simulink library "ddm"  (R2021b)
settings: Solver=VariableStepAuto  StartTime=0.0  StopTime=10.0  RelTol=1e-3
undefined symbols (not defined in the file or in its folder): ENUM_ADASACCSTA_ERROR, ENUM_ADASACCSTA_OFF, ENUM_ADASACCSTA_STANDBY, ENUM_ADASISASTA_OFF, ENUM_ALLOWMOV_ALLOWREADY, ENUM_APS, ENUM_BRKSTA_ERROR, ENUM_BRKSTA_OFF, ENUM_BRKSTA_ON, ENUM_BRKSW_INVALID, ENUM_BRKSW_OFF, ENUM_BRKSW_ON, ENUM_CHGPREACTERRSTA_OBCPRE, ENUM_DCDCFAULTSTA_ANYFAULTLV1, ENUM_DCDCFAULTSTA_ANYFAULTLV2, ENUM_DRIVETRAIN_AWD, ENUM_DRIVETRAIN_FWD, ENUM_DRIVETRAIN_RWD, ENUM_DRSEATSTA_INVALID, ENUM_EDUDRTSTA_NORMAL, ENUM_EPBSTA_APPLIED, ENUM_EPBSTA_RELEASED, ENUM_HVBATTREADYPRE_READY, ENUM_MCUWARN_LV0, ENUM_MCUWARN_LV1, ENUM_MCUWARN_LV2, ENUM_MCUWARN_LV3, ENUM_MCUWARN_NOERROR, ENUM_OBCFAULTSTA_ANYFAULT, ENUM_PAS_R2F2, ENUM_PDFAULT_BATTPDFAIL, ENUM_PDFAULT_DCDCDISABLE, ENUM_PDFAULT_MCUDISABLE, ENUM_PDFAULT_MCUDISCHRG, ENUM_POWERSTA_OFF, ENUM_POWERSTA_ON, ENUM_POWERSTA_READY, ENUM_POWERSTA_STANDBY, ENUM_PRESSINDI_LOW, ENUM_PUFAULT_BATTUPFAIL, ENUM_PUFAULT_DCDCENABLEFAIL, ENUM_PUFAULT_PRECHRGCHKFAIL, ENUM_PUFAULT_SAFETYCHKFAIL, ENUM_PUSTATE_COMPLETED, ENUM_PWRSTASW_OFF, ENUM_PWRSTASW_OFFA, ENUM_PWRSTASW_OFFCHVCHRG, ENUM_PWRSTASW_OFFCLVCHRG, ENUM_PWRSTASW_ON, ENUM_PWRSTASW_ONHVCHRG, ENUM_PWRSTASW_READY, ENUM_PWRSTASW_STANDBY, ENUM_RANGESTA_12IN, ENUM_SHIFTCOMMAND_D, ENUM_SHIFTCOMMAND_N, ENUM_SHIFTCOMMAND_P, ENUM_SHIFTCOMMAND_R, ENUM_VEHMALFUNLV_2ND, ENUM_VEHMALFUNLV_3RD, ENUM_VEHMALFUNLV_4TH ... (+835)
libraries: hcu_lib x750, $bdroot x12, simulink x5
(part 21 of 28)

== system ddm/DDM/DDM/PMM/power up and power down/BMS ready fail ==
  note: Diagnostics and Fault Handling
  note: Release Condition After Failure Decision
  note: Test Detection Criteria
  note: Test Pass Criteria
  note: Release Condition During Failure Detection
  note: Fail Safe Operation During Failure Detection
  note: Fail Safe Operation After Failure Decision
  task_time_s : Inport
  VPMM_PowerSta_enum : Inport  Port=2
  VPMM_PwrStaSW_enum : Inport  Port=3
  VINP_BMSREADY_flg : Inport  Port=4
  VPMM_PowerUpFault_enum : Inport  Port=5
  DTC_clear_request : Inport  Port=6
  VPMM_PowerUpState_enum : Inport  Port=7
  Constant : Constant  Value=ENUM_PUFAULT_BATTUPFAIL
  Constant1 : Constant  Value=ENUM_PWRSTASW_OFF
  Constant10 : Constant  Value=KDDM_BMSRdyDTC_cnt
  Constant11 : Constant  Value=KDDM_BMSRdyPassSW_flg
  Constant15 : Constant  Value=KDDM_BMSRdyCFSSW_flg
  Constant16 : Constant  Value=TRUE
  Constant19 : Constant  Value=ENUM_POWERSTA_OFF
  Constant2 : Constant  Value=ENUM_PUSTATE_COMPLETED
  Constant20 : Constant  Value=KDDM_BMSRdyDFSSW_flg
  Constant{3,21,25,27} (4 alike) : Constant  Value=FALSE
  Constant23 : Constant  Value=TRUE
  Constant24 : Constant  Value=TRUE
  Constant38 : Constant  Commented=on  Value=KDDM_BMSRdyDetTO_s
  Constant40 : Constant  Commented=on  Value=KDDM_BMSRdyDTC_cnt
  Constant43 : Constant  Value=KDDM_BMSRdyPassTO_s
  Constant44 : Constant  Value=KDDM_BMSRdyDetSW_flg
  Constant8 : Constant  Value=KDDM_BMSRdyPassTO_s
  DTC_Couter : hcu_lib/Basic_Blocks/DTC_Couter
  DTC_Info : hcu_lib/Basic_Blocks/DTC_Info
  Data Type Conversion1 : DataTypeConversion  OutDataTypeStr=uint8
  Equal : RelationalOperator  Operator=~=  OutDataTypeStr=boolean  RndMeth=Simplest
  Equal1 : RelationalOperator  Operator===  OutDataTypeStr=boolean  RndMeth=Simplest
  Equal2 : RelationalOperator  Operator===  OutDataTypeStr=boolean  RndMeth=Simplest
  Equal5 : RelationalOperator  OutDataTypeStr=boolean  RndMeth=Simplest
  Equal6 : RelationalOperator  Operator===  OutDataTypeStr=boolean  RndMeth=Simplest
  From48 : From  Commented=on  GotoTag=task_time_s
  Goto24 : Goto  Commented=on  GotoTag=VDDM_EDriveSysErrVCUErr_flg
  Logical Operator1 : Logic  Operator=OR  AllPortsSameDT=off  OutDataTypeStr=boolean
  Logical Operator{5,12,15,18} (4 alike) : Logic  AllPortsSameDT=off  OutDataTypeStr=boolean
  Logical Operator19 : Logic  Inputs=3  AllPortsSameDT=off  OutDataTypeStr=boolean
  Logical Operator2 : Logic  Operator=NOT  AllPortsSameDT=off  OutDataTypeStr=boolean
  Logical Operator3 : Logic  Operator=OR  Inputs=3  AllPortsSameDT=off  OutDataTypeStr=boolean
  Logical Operator4 : Logic  Operator=NOT  AllPortsSameDT=off  OutDataTypeStr=boolean
  Logical Operator6 : Logic  Operator=NOT  AllPortsSameDT=off  OutDataTypeStr=boolean
  Logical Operator7 : Logic  Operator=OR  AllPortsSameDT=off  OutDataTypeStr=boolean
  Logical Operator8 : Logic  Operator=OR  AllPortsSameDT=off  OutDataTypeStr=boolean
  Relay : Relay  OnSwitchValue=ONE_INT  OffSwitchValue=ZERO_INT
  SR_Latch1 : Subsystem  mask(SR_Latch){}
      mask help: SR latch function.
  SR_Latch3 : hcu_lib/Basic_Blocks/SR_Latch
  SR_Latch4 : hcu_lib/Basic_Blocks/SR_Latch
  Switch{,2,4..5} (4 alike) : Switch  Criteria=u2 ~= 0
  Test Detection Criteria : hcu_lib/Basic_Blocks/Test Detection Criteria  Commented=on
  Timer1 : hcu_lib/Basic_Blocks/Timer
  VDDM_BMSRdyDTC_raw32 : Outport
  wires:
  [DTC_clear_request] -> Logical Operator7/2
  Logical Operator7/1 -> SR_Latch3/2
  Logical Operator1/1 -> SR_Latch4/2
  Logical Operator2/1 -> Logical Operator19/3
  [DTC_clear_request] -> Logical Operator3/3
  Logical Operator12/1 -> [VDDM_BMSRdyDFS_flg]  "VDDM_BMSRdyDFS_flg"
  Logical Operator18/1 -> [VDDM_BMSRdyCFS_flg]  "VDDM_BMSRdyCFS_flg"
  [VDDM_BMSRdyCFS_flg] -> Logical Operator7/1
  Data Type Conversion1/1 -> [VDDM_BMSRdyDTC_cnt]  "VDDM_BMSRdyDTC_cnt"
  Logical Operator15/1 -> DTC_Couter/2
  [VDDM_BMSRdyPass_flg] -> Logical Operator3/1
  [DTC_clear_request] -> Logical Operator2/1
  [VDDM_BMSRdyDet_flg] -> Logical Operator19/1
  DTC_Couter/1 -> SR_Latch4/1
  Constant20/1 -> Logical Operator12/1
  Constant15/1 -> Logical Operator18/2
  [DTC_clear_request] -> Logical Operator1/2
  Constant10/1 -> DTC_Couter/3
  Logical Operator19/1 -> DTC_Couter/1
  SR_Latch4/1 -> Logical Operator18/1
  Relay/1 -> SR_Latch3/1
  SR_Latch3/1 -> Logical Operator12/2
  Constant44/1 -> Logical Operator19/2
  [VDDM_BMSRdyCFSRls_flg] -> Logical Operator3/2
  [VDDM_BMSRdyDTC_cnt] -> Relay/1
  [VDDM_BMSRdyCFSRls_flg] -> Logical Operator1/1
  Constant11/1 -> Logical Operator15/2
  Logical Operator3/1 -> Logical Operator15/1
  DTC_Couter/2 -> Data Type Conversion1/1
  [VPMM_PowerUpState_enum] -> Equal2/1
  Constant2/1 -> Equal2/2
  Constant3/1 -> Switch2/1
  VPMM_PowerUpState_enum/1 -> [VPMM_PowerUpState_enum]
  [DTC_clear_request] -> DTC_Info/4
  Constant38/1 -> Test Detection Criteria/4
  [VDDM_BMSRdyPass_flg] -> DTC_Info/2
  [VDDM_BMSRdyDet_flg] -> DTC_Info/1
  [VDDM_BMSRdyCFS_flg] -> DTC_Info/3
  DTC_Info/1 -> VDDM_BMSRdyDTC_raw32/1  "VDDM_BMSRdyDTC_raw32"
  task_time_s/1 -> [task_time_s]
  VPMM_PwrStaSW_enum/1 -> [VPMM_PwrStaSW_enum]
  VPMM_PowerSta_enum/1 -> [VPMM_PowerSta_enum]
  Constant21/1 -> Switch/3
  Equal5/1 -> SR_Latch1/1(set)
  Switch4/1 -> [VDDM_BMSRdyCFSRls_flg]  "VDDM_BMSRdyCFSRls_flg"
  Constant8/1 -> Equal5/2
  [task_time_s] -> Timer1/3
  [VPMM_PowerSta_enum] -> Equal6/1
  Constant23/1 -> Switch2/3
  Constant16/1 -> Switch/1
  Constant1/1 -> Equal/2
  From48/1 -> Test Detection Criteria/2
  Switch/1 -> Goto24/1
  Switch5/1 -> [VDDM_BMSRdyDet_flg]  "VDDM_BMSRdyDet_flg"
  Constant24/1 -> Switch4/1
  Constant40/1 -> Test Detection Criteria/3
  Constant25/1 -> Switch4/3
  [VPMM_PwrStaSW_enum] -> Equal/1
  [VDDM_BMSRdyCFS_flg] -> Switch/2
  [DTC_clear_request] -> Logical Operator8/2
  Equal2/1 -> Switch2/2
  Equal/1 -> Switch5/2
  Logical Operator8/1 -> Switch4/2
  Logical Operator6/1 -> Timer1/1
  SR_Latch1/1(latched) -> [VDDM_BMSRdyPass_flg]  "VDDM_BMSRdyPass_flg"
  Equal6/1 -> Logical Operator8/1
  Constant27/1 -> Switch5/3
  Constant43/1 -> Timer1/4
  Constant19/1 -> Equal6/2
  [VDDM_BMSRdyChk_flg] -> Switch5/1
  Timer1/1 -> Equal5/1
  Switch2/1 -> SR_Latch1/2(reset), Timer1/2, Logical Operator6/1
  DTC_clear_request/1 -> [DTC_clear_request]
  Constant/1 -> Equal1/2
  Equal1/1 -> Logical Operator5/2
  Logical Operator4/1 -> Logical Operator5/1
  VINP_BMSREADY_flg/1 -> Logical Operator4/1
  VPMM_PowerUpFault_enum/1 -> Equal1/1
  Logical Operator5/1 -> [VDDM_BMSRdyChk_flg]

== system ddm/DDM/DDM/PMM/power up and power down/DCDC disable fail ==
  note: Diagnostics and Fault Handling
  note: Test Pass Criteria
  note: Test Detection Criteria
  note: Release Condition During Failure Detection
  note: Release Condition After Failure Decision
  note: Fail Safe Operation During Failure Detection
  note: Fail Safe Operation After Failure Decision
  task_time_s : Inport
  VPMM_PowerSta_enum : Inport  Port=2
  VPMM_PwrStaSW_enum : Inport  Port=3
  VPMM_PowerDownFault_enum : Inport  Port=4
  DTC_clear_request : Inport  Port=5
  Constant : Constant  Value=ENUM_PDFAULT_DCDCDISABLE
  Constant1 : Constant  Value=ENUM_PWRSTASW_OFF
  Constant10 : Constant  Value=KDDM_DCDCDisDTC_cnt
  Constant11 : Constant  Value=KDDM_DCDCDisPassSW_flg
  Constant15 : Constant  Value=KDDM_DCDCDisCFSSW_flg
  Constant16 : Constant  Value=TRUE
  Constant17 : Constant  Value=KDDM_DCDCDisPassTO_s
  Constant19 : Constant  Value=ENUM_POWERSTA_OFF
  Constant20 : Constant  Value=KDDM_DCDCDisDFSSW_flg
  Constant21 : Constant  Value=FALSE
  Constant22 : Constant  Value=ENUM_PWRSTASW_OFF
  Constant23 : Constant  Value=TRUE
  Constant24 : Constant  Value=TRUE
  Constant25 : Constant  Value=FALSE
  Constant27 : Constant  Value=FALSE
  Constant38 : Constant  Commented=on  Value=KDDM_DCDCDisDetTO_s
  Constant40 : Constant  Commented=on  Value=KDDM_DCDCDisDTC_cnt
  Constant43 : Constant  Value=KDDM_DCDCDisPassTO_s
  Constant44 : Constant  Value=KDDM_DCDCDisDetSW_flg
  DTC_Couter : hcu_lib/Basic_Blocks/DTC_Couter
  DTC_Info : hcu_lib/Basic_Blocks/DTC_Info
  Data Type Conversion1 : DataTypeConversion  OutDataTypeStr=uint8
  Equal1 : RelationalOperator  Operator===  OutDataTypeStr=boolean  RndMeth=Simplest
  Equal2 : RelationalOperator  Operator=~=  OutDataTypeStr=boolean  RndMeth=Simplest
  Equal4 : RelationalOperator  Operator=~=  OutDataTypeStr=boolean  RndMeth=Simplest
  Equal6 : RelationalOperator  OutDataTypeStr=boolean  RndMeth=Simplest
  Equal7 : RelationalOperator  Operator===  OutDataTypeStr=boolean  RndMeth=Simplest
  From48 : From  Commented=on  GotoTag=task_time_s
  Goto24 : Goto  Commented=on  GotoTag=VDDM_EDriveSysErrVCUErr_flg
  Logical Operator1 : Logic  Operator=NOT  AllPortsSameDT=off  OutDataTypeStr=boolean
  Logical Operator12 : Logic  AllPortsSameDT=off  OutDataTypeStr=boolean
  Logical Operator15 : Logic  AllPortsSameDT=off  OutDataTypeStr=boolean
  Logical Operator18 : Logic  AllPortsSameDT=off  OutDataTypeStr=boolean
  Logical Operator19 : Logic  Inputs=3  AllPortsSameDT=off  OutDataTypeStr=boolean
  Logical Operator2 : Logic  Operator=OR  AllPortsSameDT=off  OutDataTypeStr=boolean
  Logical Operator3 : Logic  Operator=OR  Inputs=3  AllPortsSameDT=off  OutDataTypeStr=boolean
  Logical Operator4 : Logic  Operator=OR  AllPortsSameDT=off  OutDataTypeStr=boolean
  Logical Operator6 : Logic  Operator=NOT  AllPortsSameDT=off  OutDataTypeStr=boolean
  Logical Operator8 : Logic  Operator=OR  AllPortsSameDT=off  OutDataTypeStr=boolean
  Relay : Relay  OnSwitchValue=ONE_INT  OffSwitchValue=ZERO_INT
  SR_Latch1 : Subsystem  mask(SR_Latch){}
      mask help: SR latch function.
  SR_Latch3 : hcu_lib/Basic_Blocks/SR_Latch
  SR_Latch4 : hcu_lib/Basic_Blocks/SR_Latch
  Switch{,1,4..5} (4 alike) : Switch  Criteria=u2 ~= 0
  Test Detection Criteria : hcu_lib/Basic_Blocks/Test Detection Criteria  Commented=on
  Timer1 : hcu_lib/Basic_Blocks/Timer
  VDDM_DCDCDisDTC_raw32 : Outport
  wires:
  [VDDM_DCDCDisDet_flg] -> Logical Operator19/1
  [DTC_clear_request] -> Logical Operator3/3
  DTC_Couter/2 -> Data Type Conversion1/1
  Logical Operator2/1 -> SR_Latch4/2
  Logical Operator1/1 -> Logical Operator19/3
  [DTC_clear_request] -> Logical Operator1/1
  Relay/1 -> SR_Latch3/1
  Constant20/1 -> Logical Operator12/1
  [VDDM_DCDCDisCFSRls_flg] -> Logical Operator2/1
  SR_Latch4/1 -> Logical Operator18/1
  [VDDM_DCDCDisCFS_flg] -> Logical Operator4/1
  [VDDM_DCDCDisDTC_cnt] -> Relay/1
  Logical Operator3/1 -> Logical Operator15/1
  Logical Operator18/1 -> [VDDM_DCDCDisCFS_flg]  "VDDM_DCDCDisCFS_flg"
  Constant11/1 -> Logical Operator15/2
  Constant10/1 -> DTC_Couter/3
  [VDDM_DCDCDisPass_flg] -> Logical Operator3/1
  [DTC_clear_request] -> Logical Operator4/2
  Constant44/1 -> Logical Operator19/2
  Logical Operator15/1 -> DTC_Couter/2
  [DTC_clear_request] -> Logical Operator2/2
  SR_Latch3/1 -> Logical Operator12/2
  [VDDM_DCDCDisCFSRls_flg] -> Logical Operator3/2
  Logical Operator19/1 -> DTC_Couter/1
  Logical Operator12/1 -> [VDDM_DCDCDisDFS_flg]  "VDDM_DCDCDisDFS_flg"
  Constant15/1 -> Logical Operator18/2
  Data Type Conversion1/1 -> [VDDM_DCDCDisDTC_cnt]  "VDDM_DCDCDisDTC_cnt"
  DTC_Couter/1 -> SR_Latch4/1
  Logical Operator4/1 -> SR_Latch3/2
  [DTC_clear_request] -> DTC_Info/4
  Constant38/1 -> Test Detection Criteria/4
  [VDDM_DCDCDisDet_flg] -> DTC_Info/1
  [VDDM_DCDCDisCFS_flg] -> DTC_Info/3
  [VDDM_DCDCDisPass_flg] -> DTC_Info/2
  DTC_Info/1 -> VDDM_DCDCDisDTC_raw32/1  "VDDM_DCDCDisDTC_raw32"
  Equal1/1 -> [VDDM_DCDCDisChk_flg]
  DTC_clear_request/1 -> [DTC_clear_request]
  Constant/1 -> Equal1/2
  VPMM_PowerDownFault_enum/1 -> Equal1/1
  Equal7/1 -> Logical Operator8/1
  Constant1/1 -> Equal2/2
  [VPMM_PwrStaSW_enum] -> Equal2/1
  Constant40/1 -> Test Detection Criteria/3
  [DTC_clear_request] -> Logical Operator8/2
  Timer1/1 -> Equal6/1
  [task_time_s] -> Timer1/3
  Constant22/1 -> Equal4/2
  Switch1/1 -> Timer1/2, SR_Latch1/2(reset), Logical Operator6/1
  Equal2/1 -> Switch1/2
  Equal4/1 -> Switch5/2
  [VPMM_PowerSta_enum] -> Equal7/1
  SR_Latch1/1(latched) -> [VDDM_DCDCDisPass_flg]  "VDDM_DCDCDisPass_flg"
  Constant23/1 -> Switch1/3
  [VDDM_DCDCDisChk_flg] -> Switch1/1
  [VPMM_PwrStaSW_enum] -> Equal4/1
  Constant43/1 -> Timer1/4
  Equal6/1 -> SR_Latch1/1(set)
  Constant17/1 -> Equal6/2
  Constant27/1 -> Switch5/3
  Constant25/1 -> Switch4/3
  Switch4/1 -> [VDDM_DCDCDisCFSRls_flg]  "VDDM_DCDCDisCFSRls_flg"
  Constant16/1 -> Switch/1
  [VDDM_DCDCDisCFS_flg] -> Switch/2
  [VDDM_DCDCDisChk_flg] -> Switch5/1
  Constant19/1 -> Equal7/2
  Constant21/1 -> Switch/3
  Constant24/1 -> Switch4/1
  From48/1 -> Test Detection Criteria/2
  Switch/1 -> Goto24/1
  Logical Operator8/1 -> Switch4/2
  Logical Operator6/1 -> Timer1/1
  Switch5/1 -> [VDDM_DCDCDisDet_flg]  "VDDM_DCDCDisDet_flg"
  task_time_s/1 -> [task_time_s]
  VPMM_PwrStaSW_enum/1 -> [VPMM_PwrStaSW_enum]
  VPMM_PowerSta_enum/1 -> [VPMM_PowerSta_enum]

== system ddm/DDM/DDM/PMM/power up and power down/DCDC enable fail ==
  note: Diagnostics and Fault Handling
  note: Fail Safe Operation After Failure Decision
  note: Fail Safe Operation During Failure Detection
  note: Release Condition During Failure Detection
  note: Test Pass Criteria
  note: Test Detection Criteria
  note: Release Condition After Failure Decision
  task_time_s : Inport
  VPMM_PowerSta_enum : Inport  Port=2
  VPMM_PwrStaSW_enum : Inport  Port=3
  VINP_DCDCEnabled_flg : Inport  Port=4
  VPMM_PowerUpFault_enum : Inport  Port=5
  DTC_clear_request : Inport  Port=6
  VPMM_PowerUpState_enum : Inport  Port=7
  Constant : Constant  Value=ENUM_PUFAULT_DCDCENABLEFAIL
  Constant1 : Constant  Value=ENUM_PUSTATE_COMPLETED
  Constant10 : Constant  Value=KDDM_DCDCEnaDTC_cnt
  Constant11 : Constant  Value=KDDM_DCDCEnaPassSW_flg
  Constant15 : Constant  Value=KDDM_DCDCEnaCFSSW_flg
  Constant16 : Constant  Value=TRUE
  Constant19 : Constant  Value=ENUM_POWERSTA_OFF
  Constant{2,21,25,27} (4 alike) : Constant  Value=FALSE
  Constant20 : Constant  Value=KDDM_DCDCEnaDFSSW_flg
  Constant23 : Constant  Value=TRUE
  Constant24 : Constant  Value=TRUE
  Constant26 : Constant  Value=ENUM_PWRSTASW_OFF
  Constant38 : Constant  Commented=on  Value=KDDM_DCDCEnaDetTO_s
  Constant40 : Constant  Commented=on  Value=KDDM_DCDCEnaDTC_cnt
  Constant43 : Constant  Value=KDDM_DCDCEnaPassTO_s
  Constant44 : Constant  Value=KDDM_DCDCEnaDetSW_flg
  Constant8 : Constant  Value=KDDM_DCDCEnaPassTO_s
  DTC_Couter : hcu_lib/Basic_Blocks/DTC_Couter
  DTC_Info : hcu_lib/Basic_Blocks/DTC_Info
  Data Type Conversion1 : DataTypeConversion  OutDataTypeStr=uint8
  Equal : RelationalOperator  Operator=~=  OutDataTypeStr=boolean  RndMeth=Simplest
  Equal1 : RelationalOperator  Operator===  OutDataTypeStr=boolean  RndMeth=Simplest
  Equal2 : RelationalOperator  Operator===  OutDataTypeStr=boolean  RndMeth=Simplest
  Equal5 : RelationalOperator  OutDataTypeStr=boolean  RndMeth=Simplest
  Equal6 : RelationalOperator  Operator===  OutDataTypeStr=boolean  RndMeth=Simplest
  From48 : From  Commented=on  GotoTag=task_time_s
  Goto24 : Goto  Commented=on  GotoTag=VDDM_EDriveSysErrVCUErr_flg
  Logical Operator1 : Logic  Operator=NOT  AllPortsSameDT=off  OutDataTypeStr=boolean
  Logical Operator{5,12,15,18} (4 alike) : Logic  AllPortsSameDT=off  OutDataTypeStr=boolean
  Logical Operator19 : Logic  Inputs=3  AllPortsSameDT=off  OutDataTypeStr=boolean
  Logical Operator2 : Logic  Operator=OR  AllPortsSameDT=off  OutDataTypeStr=boolean
  Logical Operator3 : Logic  Operator=OR  Inputs=3  AllPortsSameDT=off  OutDataTypeStr=boolean
  Logical Operator4 : Logic  Operator=NOT  AllPortsSameDT=off  OutDataTypeStr=boolean
  Logical Operator6 : Logic  Operator=NOT  AllPortsSameDT=off  OutDataTypeStr=boolean
  Logical Operator7 : Logic  Operator=OR  AllPortsSameDT=off  OutDataTypeStr=boolean
  Logical Operator8 : Logic  Operator=OR  AllPortsSameDT=off  OutDataTypeStr=boolean
  Relay : Relay  OnSwitchValue=ONE_INT  OffSwitchValue=ZERO_INT
  SR_Latch1 : Subsystem  mask(SR_Latch){}
      mask help: SR latch function.
  SR_Latch3 : hcu_lib/Basic_Blocks/SR_Latch
  SR_Latch4 : hcu_lib/Basic_Blocks/SR_Latch
  Switch{,2,4..5} (4 alike) : Switch  Criteria=u2 ~= 0
  Test Detection Criteria : hcu_lib/Basic_Blocks/Test Detection Criteria  Commented=on
  Timer1 : hcu_lib/Basic_Blocks/Timer
  VDDM_DCDCEnaDTC_raw32 : Outport
  wires:
  [DTC_clear_request] -> Logical Operator1/1
  Logical Operator7/1 -> SR_Latch3/2
  Logical Operator1/1 -> Logical Operator19/3
  [DTC_clear_request] -> Logical Operator3/3
  Constant20/1 -> Logical Operator12/1
  [VDDM_DCDCEnaCFS_flg] -> Logical Operator7/1
  Constant44/1 -> Logical Operator19/2
  Constant11/1 -> Logical Operator15/2
  [VDDM_DCDCEnaDTC_cnt] -> Relay/1
  [DTC_clear_request] -> Logical Operator2/2
  SR_Latch3/1 -> Logical Operator12/2
  Relay/1 -> SR_Latch3/1
  SR_Latch4/1 -> Logical Operator18/1
  [VDDM_DCDCEnaCFSRls_flg] -> Logical Operator3/2
  Logical Operator15/1 -> DTC_Couter/2
  Constant15/1 -> Logical Operator18/2
  [DTC_clear_request] -> Logical Operator7/2
  [VDDM_DCDCEnaPass_flg] -> Logical Operator3/1
  Logical Operator12/1 -> [VDDM_DCDCEnaDFS_flg]  "VDDM_DCDCEnaDFS_flg"
  Logical Operator19/1 -> DTC_Couter/1
  Constant10/1 -> DTC_Couter/3
  DTC_Couter/1 -> SR_Latch4/1
  [VDDM_DCDCEnaDet_flg] -> Logical Operator19/1
  Logical Operator2/1 -> SR_Latch4/2
  DTC_Couter/2 -> Data Type Conversion1/1
  Data Type Conversion1/1 -> [VDDM_DCDCEnaDTC_cnt]  "VDDM_DCDCEnaDTC_cnt"
  Logical Operator18/1 -> [VDDM_DCDCEnaCFS_flg]  "VDDM_DCDCEnaCFS_flg"
  [VDDM_DCDCEnaCFSRls_flg] -> Logical Operator2/1
  Logical Operator3/1 -> Logical Operator15/1
  [VPMM_PowerUpState_enum] -> Equal2/1
  Constant1/1 -> Equal2/2
  Constant2/1 -> Switch2/1
  VPMM_PowerUpState_enum/1 -> [VPMM_PowerUpState_enum]
  [DTC_clear_request] -> DTC_Info/4
  Constant38/1 -> Test Detection Criteria/4
  [VDDM_DCDCEnaDet_flg] -> DTC_Info/1
  [VDDM_DCDCEnaCFS_flg] -> DTC_Info/3
  [VDDM_DCDCEnaPass_flg] -> DTC_Info/2
  DTC_Info/1 -> VDDM_DCDCEnaDTC_raw32/1  "VDDM_DCDCEnaDTC_raw32"
  Logical Operator5/1 -> [VDDM_DCDCEnaChk_flg]
  VPMM_PowerUpFault_enum/1 -> Equal1/1
  VINP_DCDCEnabled_flg/1 -> Logical Operator4/1
  Logical Operator4/1 -> Logical Operator5/1
  Equal1/1 -> Logical Operator5/2
  Constant/1 -> Equal1/2
  DTC_clear_request/1 -> [DTC_clear_request]
  Switch2/1 -> Logical Operator6/1, Timer1/2, SR_Latch1/2(reset)
  Timer1/1 -> Equal5/1
  [VDDM_DCDCEnaChk_flg] -> Switch5/1
  Constant19/1 -> Equal6/2
  Constant43/1 -> Timer1/4
  Constant27/1 -> Switch5/3
  Equal6/1 -> Logical Operator8/1
  SR_Latch1/1(latched) -> [VDDM_DCDCEnaPass_flg]  "VDDM_DCDCEnaPass_flg"
  Logical Operator6/1 -> Timer1/1
  Logical Operator8/1 -> Switch4/2
  Equal/1 -> Switch5/2
  Equal2/1 -> Switch2/2
  [DTC_clear_request] -> Logical Operator8/2
  [VDDM_DCDCEnaCFS_flg] -> Switch/2
  [VPMM_PwrStaSW_enum] -> Equal/1
  Constant25/1 -> Switch4/3
  Constant40/1 -> Test Detection Criteria/3
  Constant24/1 -> Switch4/1
  Switch5/1 -> [VDDM_DCDCEnaDet_flg]  "VDDM_DCDCEnaDet_flg"
  Switch/1 -> Goto24/1
  From48/1 -> Test Detection Criteria/2
  Constant26/1 -> Equal/2
  Constant16/1 -> Switch/1
  Constant23/1 -> Switch2/3
  [VPMM_PowerSta_enum] -> Equal6/1
  [task_time_s] -> Timer1/3
  Constant8/1 -> Equal5/2
  Switch4/1 -> [VDDM_DCDCEnaCFSRls_flg]  "VDDM_DCDCEnaCFSRls_flg"
  Equal5/1 -> SR_Latch1/1(set)
  Constant21/1 -> Switch/3
  VPMM_PowerSta_enum/1 -> [VPMM_PowerSta_enum]
  VPMM_PwrStaSW_enum/1 -> [VPMM_PwrStaSW_enum]
  task_time_s/1 -> [task_time_s]

== system ddm/DDM/DDM/PMM/power up and power down/DCDC ready for precharge fail ==
  note: Diagnostics and Fault Handling
  note: Fail Safe Operation During Failure Detection
  note: Fail Safe Operation After Failure Decision
  note: Test Pass Criteria
  note: Release Condition After Failure Decision
  note: Test Detection Criteria
  note: Release Condition During Failure Detection
  task_time_s : Inport
  VPMM_PowerSta_enum : Inport  Port=2
  VPMM_PwrStaSW_enum : Inport  Port=3
  VINP_DCDCReady4Pre_flg : Inport  Port=4
  VPMM_PowerUpFault_enum : Inport  Port=5
  VINP_ReqClrDTC_flg : Inport  Port=6
  VPMM_PowerUpState_enum : Inport  Port=7
  Constant : Constant  Value=ENUM_PUFAULT_PRECHRGCHKFAIL
  Constant1 : Constant  Value=ENUM_PUSTATE_COMPLETED
  Constant10 : Constant  Value=KDDM_DCDC4PreDTC_cnt
  Constant11 : Constant  Value=KDDM_DCDC4PrePassSW_flg
  Constant15 : Constant  Value=KDDM_DCDC4PreCFSSW_flg
  Constant16 : Constant  Value=TRUE
  Constant19 : Constant  Value=ENUM_POWERSTA_OFF
  Constant{2,21,25,27} (4 alike) : Constant  Value=FALSE
  Constant20 : Constant  Value=KDDM_DCDC4PreDFSSW_flg
  Constant23 : Constant  Value=TRUE
  Constant24 : Constant  Value=TRUE
  Constant26 : Constant  Value=ENUM_PWRSTASW_OFF
  Constant38 : Constant  Commented=on  Value=KDDM_DCDC4PreDetTO_s
  Constant40 : Constant  Commented=on  Value=KDDM_DCDC4PreDTC_cnt
  Constant43 : Constant  Value=KDDM_DCDC4PrePassTO_s
  Constant44 : Constant  Value=KDDM_DCDC4PreDetSW_flg
  Constant8 : Constant  Value=KDDM_DCDC4PrePassTO_s
  DTC_Couter : hcu_lib/Basic_Blocks/DTC_Couter
  DTC_Info : hcu_lib/Basic_Blocks/DTC_Info
  Data Type Conversion1 : DataTypeConversion  OutDataTypeStr=uint8
  Equal : RelationalOperator  Operator=~=  OutDataTypeStr=boolean  RndMeth=Simplest
  Equal1 : RelationalOperator  Operator===  OutDataTypeStr=boolean  RndMeth=Simplest
  Equal2 : RelationalOperator  Operator===  OutDataTypeStr=boolean  RndMeth=Simplest
  Equal5 : RelationalOperator  OutDataTypeStr=boolean  RndMeth=Simplest
  Equal6 : RelationalOperator  Operator===  OutDataTypeStr=boolean  RndMeth=Simplest
  From48 : From  Commented=on  GotoTag=task_time_s
  Goto24 : Goto  Commented=on  GotoTag=VDDM_EDriveSysErrVCUErr_flg
  Logical Operator1 : Logic  Operator=NOT  AllPortsSameDT=off  OutDataTypeStr=boolean
  Logical Operator{5,12,15,18} (4 alike) : Logic  AllPortsSameDT=off  OutDataTypeStr=boolean
  Logical Operator19 : Logic  Inputs=3  AllPortsSameDT=off  OutDataTypeStr=boolean
  Logical Operator2 : Logic  Operator=OR  AllPortsSameDT=off  OutDataTypeStr=boolean
  Logical Operator3 : Logic  Operator=OR  Inputs=3  AllPortsSameDT=off  OutDataTypeStr=boolean
  Logical Operator4 : Logic  Operator=NOT  AllPortsSameDT=off  OutDataTypeStr=boolean
  Logical Operator6 : Logic  Operator=NOT  AllPortsSameDT=off  OutDataTypeStr=boolean
  Logical Operator7 : Logic  Operator=OR  AllPortsSameDT=off  OutDataTypeStr=boolean
  Logical Operator8 : Logic  Operator=OR  AllPortsSameDT=off  OutDataTypeStr=boolean
  Relay : Relay  OnSwitchValue=ONE_INT  OffSwitchValue=ZERO_INT
  SR_Latch1 : Subsystem  mask(SR_Latch){}
      mask help: SR latch function.
  SR_Latch3 : hcu_lib/Basic_Blocks/SR_Latch
  SR_Latch4 : hcu_lib/Basic_Blocks/SR_Latch
  Switch{,2,4..5} (4 alike) : Switch  Criteria=u2 ~= 0
  Test Detection Criteria : hcu_lib/Basic_Blocks/Test Detection Criteria  Commented=on
  Timer1 : hcu_lib/Basic_Blocks/Timer
  VDDM_DCDC4PreDTC_raw32 : Outport
  wires:
  Logical Operator7/1 -> SR_Latch3/2
  [DTC_clear_request] -> Logical Operator7/2
  Constant11/1 -> Logical Operator15/2
  [DTC_clear_request] -> Logical Operator2/2
  Relay/1 -> SR_Latch3/1
  Logical Operator2/1 -> SR_Latch4/2
  [DTC_clear_request] -> Logical Operator3/3
  SR_Latch4/1 -> Logical Operator18/1
  Logical Operator1/1 -> Logical Operator19/3
  [VDDM_DCDC4PreCFS_flg] -> Logical Operator7/1
  Data Type Conversion1/1 -> [VDDM_DCDC4PreDTC_cnt]  "VDDM_DCDC4PreDTC_cnt"
  DTC_Couter/1 -> SR_Latch4/1
  [DTC_clear_request] -> Logical Operator1/1
  Constant20/1 -> Logical Operator12/1
  Logical Operator18/1 -> [VDDM_DCDC4PreCFS_flg]  "VDDM_DCDC4PreCFS_flg"
  Logical Operator19/1 -> DTC_Couter/1
  [VDDM_DCDC4PrePass_flg] -> Logical Operator3/1
  [VDDM_DCDC4PreCFSRls_flg] -> Logical Operator2/1
  Constant15/1 -> Logical Operator18/2
  Logical Operator12/1 -> [VDDM_DCDC4PreDFS_flg]  "VDDM_DCDC4PreDFS_flg"
  Logical Operator3/1 -> Logical Operator15/1
  SR_Latch3/1 -> Logical Operator12/2
  DTC_Couter/2 -> Data Type Conversion1/1
  Constant10/1 -> DTC_Couter/3
  [VDDM_DCDC4PreDTC_cnt] -> Relay/1
  Constant44/1 -> Logical Operator19/2
  Logical Operator15/1 -> DTC_Couter/2
  [VDDM_DCDC4PreCFSRls_flg] -> Logical Operator3/2
  [VDDM_DCDC4PreDet_flg] -> Logical Operator19/1
  [VPMM_PowerUpState_enum] -> Equal2/1
  Constant1/1 -> Equal2/2
  Constant2/1 -> Switch2/1
  VPMM_PowerUpState_enum/1 -> [VPMM_PowerUpState_enum]
  [DTC_clear_request] -> DTC_Info/4
  Constant38/1 -> Test Detection Criteria/4
  [VDDM_DCDC4PreDet_flg] -> DTC_Info/1
  [VDDM_DCDC4PreCFS_flg] -> DTC_Info/3
  [VDDM_DCDC4PrePass_flg] -> DTC_Info/2
  DTC_Info/1 -> VDDM_DCDC4PreDTC_raw32/1  "VDDM_DCDC4PreDTC_raw32"
  Logical Operator4/1 -> Logical Operator5/1
  VINP_DCDCReady4Pre_flg/1 -> Logical Operator4/1
  Logical Operator5/1 -> [VDDM_DCDC4PreChk_flg]
  VPMM_PowerUpFault_enum/1 -> Equal1/1
  Constant/1 -> Equal1/2
  Equal1/1 -> Logical Operator5/2
  VINP_ReqClrDTC_flg/1 -> [DTC_clear_request]
  Switch4/1 -> [VDDM_DCDC4PreCFSRls_flg]  "VDDM_DCDC4PreCFSRls_flg"
  Constant21/1 -> Switch/3
  Equal5/1 -> SR_Latch1/1(set)
  Constant8/1 -> Equal5/2
  [task_time_s] -> Timer1/3
  Equal2/1 -> Switch2/2
  From48/1 -> Test Detection Criteria/2
  [VPMM_PowerSta_enum] -> Equal6/1
  Switch/1 -> Goto24/1
  Constant26/1 -> Equal/2
  Constant23/1 -> Switch2/3
  Constant16/1 -> Switch/1
  Constant24/1 -> Switch4/1
  Constant25/1 -> Switch4/3
  Constant43/1 -> Timer1/4
  Constant40/1 -> Test Detection Criteria/3
  [VPMM_PwrStaSW_enum] -> Equal/1
  Switch5/1 -> [VDDM_DCDC4PreDet_flg]  "VDDM_DCDC4PreDet_flg"
  [VDDM_DCDC4PreCFS_flg] -> Switch/2
  [DTC_clear_request] -> Logical Operator8/2
  Equal/1 -> Switch5/2
  Logical Operator8/1 -> Switch4/2
  Constant27/1 -> Switch5/3
  Logical Operator6/1 -> Timer1/1
  Constant19/1 -> Equal6/2
  SR_Latch1/1(latched) -> [VDDM_DCDC4PrePass_flg]  "VDDM_DCDC4PrePass_flg"
  Timer1/1 -> Equal5/1
  Equal6/1 -> Logical Operator8/1
  [VDDM_DCDC4PreChk_flg] -> Switch5/1
  Switch2/1 -> Logical Operator6/1, Timer1/2, SR_Latch1/2(reset)
  task_time_s/1 -> [task_time_s]
  VPMM_PwrStaSW_enum/1 -> [VPMM_PwrStaSW_enum]
  VPMM_PowerSta_enum/1 -> [VPMM_PowerSta_enum]

== system ddm/DDM/DDM/PMM/power up and power down/HVB ready for precharge fail ==
  note: Diagnostics and Fault Handling
  note: Release Condition During Failure Detection
  note: Test Detection Criteria
  note: Test Pass Criteria
  note: Fail Safe Operation During Failure Detection
  note: Release Condition After Failure Decision
  note: Fail Safe Operation After Failure Decision
  task_time_s : Inport
  VPMM_PowerSta_enum : Inport  Port=2
  VPMM_PwrStaSW_enum : Inport  Port=3
  VINP_HVBattReady4Pre_enum : Inport  Port=4
  VPMM_PowerUpFault_enum : Inport  Port=5
  DTC_clear_request : Inport  Port=6
  VPMM_PowerUpState_enum : Inport  Port=7
  Constant : Constant  Value=ENUM_PUFAULT_PRECHRGCHKFAIL
  Constant1 : Constant  Value=ENUM_PUSTATE_COMPLETED
  Constant10 : Constant  Value=KDDM_HVB4PreDTC_cnt
  Constant11 : Constant  Value=KDDM_HVB4PrePassSW_flg
  Constant15 : Constant  Value=KDDM_HVB4PreCFSSW_flg
  Constant16 : Constant  Value=TRUE
  Constant19 : Constant  Value=ENUM_POWERSTA_OFF
  Constant{2,21,25,27} (4 alike) : Constant  Value=FALSE
  Constant20 : Constant  Value=KDDM_HVB4PreDFSSW_flg
  Constant23 : Constant  Value=TRUE
  Constant24 : Constant  Value=TRUE
  Constant26 : Constant  Value=ENUM_PWRSTASW_OFF
  Constant3 : Constant  Value=ENUM_HVBATTREADYPRE_READY
  Constant38 : Constant  Commented=on  Value=KDDM_HVB4PreDetTO_s
  Constant40 : Constant  Commented=on  Value=KDDM_HVB4PreDTC_cnt
  Constant43 : Constant  Value=KDDM_HVB4PrePassTO_s
  Constant44 : Constant  Value=KDDM_HVB4PreDetSW_flg
  Constant8 : Constant  Value=KDDM_HVB4PrePassTO_s
  DTC_Couter : hcu_lib/Basic_Blocks/DTC_Couter
  DTC_Info : hcu_lib/Basic_Blocks/DTC_Info
  Data Type Conversion1 : DataTypeConversion  OutDataTypeStr=uint8
  Equal : RelationalOperator  Operator=~=  OutDataTypeStr=boolean  RndMeth=Simplest
  Equal1 : RelationalOperator  Operator===  OutDataTypeStr=boolean  RndMeth=Simplest
  Equal24 : RelationalOperator  Operator=~=  OutDataTypeStr=boolean  RndMeth=Simplest
  Equal4 : RelationalOperator  OutDataTypeStr=boolean  RndMeth=Simplest
  Equal5 : RelationalOperator  Operator===  OutDataTypeStr=boolean  RndMeth=Simplest
  Equal8 : RelationalOperator  Operator===  OutDataTypeStr=boolean  RndMeth=Simplest
  From48 : From  Commented=on  GotoTag=task_time_s
  Goto24 : Goto  Commented=on  GotoTag=VDDM_EDriveSysErrVCUErr_flg
  Logical Operator1 : Logic  Operator=OR  AllPortsSameDT=off  OutDataTypeStr=boolean
  Logical Operator{4,12,15,18} (4 alike) : Logic  AllPortsSameDT=off  OutDataTypeStr=boolean
  Logical Operator19 : Logic  Inputs=3  AllPortsSameDT=off  OutDataTypeStr=boolean
  Logical Operator2 : Logic  Operator=NOT  AllPortsSameDT=off  OutDataTypeStr=boolean
  Logical Operator3 : Logic  Operator=OR  Inputs=3  AllPortsSameDT=off  OutDataTypeStr=boolean
  Logical Operator5 : Logic  Operator=OR  AllPortsSameDT=off  OutDataTypeStr=boolean
  Logical Operator6 : Logic  Operator=NOT  AllPortsSameDT=off  OutDataTypeStr=boolean
  Logical Operator8 : Logic  Operator=OR  AllPortsSameDT=off  OutDataTypeStr=boolean
  Relay : Relay  OnSwitchValue=ONE_INT  OffSwitchValue=ZERO_INT
  SR_Latch1 : Subsystem  mask(SR_Latch){}
      mask help: SR latch function.
  SR_Latch3 : hcu_lib/Basic_Blocks/SR_Latch
  SR_Latch4 : hcu_lib/Basic_Blocks/SR_Latch
  Switch{,2,4..5} (4 alike) : Switch  Criteria=u2 ~= 0
  Test Detection Criteria : hcu_lib/Basic_Blocks/Test Detection Criteria  Commented=on
  Timer1 : hcu_lib/Basic_Blocks/Timer
  VDDM_HVB4PreDTC_raw32 : Outport
  wires:
  [DTC_clear_request] -> Logical Operator5/2
  [DTC_clear_request] -> Logical Operator3/3
  Logical Operator5/1 -> SR_Latch3/2
  [VDDM_HVB4PreCFSRls_flg] -> Logical Operator3/2
  [DTC_clear_request] -> Logical Operator2/1
  [DTC_clear_request] -> Logical Operator1/2
  Logical Operator2/1 -> Logical Operator19/3
  Logical Operator1/1 -> SR_Latch4/2
  [VDDM_HVB4PreCFS_flg] -> Logical Operator5/1
  Constant10/1 -> DTC_Couter/3
  [VDDM_HVB4PreCFSRls_flg] -> Logical Operator1/1
  SR_Latch3/1 -> Logical Operator12/2
  Relay/1 -> SR_Latch3/1
  DTC_Couter/1 -> SR_Latch4/1
  Constant15/1 -> Logical Operator18/2
  Logical Operator12/1 -> [VDDM_HVB4PreDFS_flg]  "VDDM_HVB4PreDFS_flg"
  Constant44/1 -> Logical Operator19/2
  DTC_Couter/2 -> Data Type Conversion1/1
  Constant20/1 -> Logical Operator12/1
  [VDDM_HVB4PreDet_flg] -> Logical Operator19/1
  Logical Operator18/1 -> [VDDM_HVB4PreCFS_flg]  "VDDM_HVB4PreCFS_flg"
  [VDDM_HVB4PreDTC_cnt] -> Relay/1
  Logical Operator3/1 -> Logical Operator15/1
  SR_Latch4/1 -> Logical Operator18/1
  Data Type Conversion1/1 -> [VDDM_HVB4PreDTC_cnt]  "VDDM_HVB4PreDTC_cnt"
  [VDDM_HVB4PrePass_flg] -> Logical Operator3/1
  Logical Operator15/1 -> DTC_Couter/2
  Constant11/1 -> Logical Operator15/2
  Logical Operator19/1 -> DTC_Couter/1
  VPMM_PowerUpState_enum/1 -> [VPMM_PowerUpState_enum]
  [DTC_clear_request] -> DTC_Info/4
  Constant38/1 -> Test Detection Criteria/4
  [VDDM_HVB4PreDet_flg] -> DTC_Info/1
  [VDDM_HVB4PrePass_flg] -> DTC_Info/2
  [VDDM_HVB4PreCFS_flg] -> DTC_Info/3
  DTC_Info/1 -> VDDM_HVB4PreDTC_raw32/1  "VDDM_HVB4PreDTC_raw32"
  Equal1/1 -> Switch2/2
  [task_time_s] -> Timer1/3
  Logical Operator4/1 -> [VDDM_HVB4PreChk_flg]
  Equal8/1 -> Logical Operator4/2
  Equal24/1 -> Logical Operator4/1
  VPMM_PowerUpFault_enum/1 -> Equal8/1
  Constant/1 -> Equal8/2
  DTC_clear_request/1 -> [DTC_clear_request]
  [VPMM_PowerUpState_enum] -> Equal1/1
  Constant2/1 -> Switch2/1
  Constant1/1 -> Equal1/2
  [VDDM_HVB4PreChk_flg] -> Switch5/1
  Equal5/1 -> Logical Operator8/1
  Timer1/1 -> Equal4/1
  Constant27/1 -> Switch5/3
  Constant19/1 -> Equal5/2
  Logical Operator6/1 -> Timer1/1
  SR_Latch1/1(latched) -> [VDDM_HVB4PrePass_flg]  "VDDM_HVB4PrePass_flg"
  Constant24/1 -> Switch4/1
  [VPMM_PwrStaSW_enum] -> Equal/1
  [VDDM_HVB4PreCFS_flg] -> Switch/2
  From48/1 -> Test Detection Criteria/2
  Equal/1 -> Switch5/2
  Switch2/1 -> Logical Operator6/1, Timer1/2, SR_Latch1/2(reset)
  Switch/1 -> Goto24/1
  [VPMM_PowerSta_enum] -> Equal5/1
  Constant16/1 -> Switch/1
  Logical Operator8/1 -> Switch4/2
  Constant26/1 -> Equal/2
  Switch4/1 -> [VDDM_HVB4PreCFSRls_flg]  "VDDM_HVB4PreCFSRls_flg"
  Equal4/1 -> SR_Latch1/1(set)
  Constant21/1 -> Switch/3
  Constant25/1 -> Switch4/3
  Constant8/1 -> Equal4/2
  Constant23/1 -> Switch2/3
  [DTC_clear_request] -> Logical Operator8/2
  Switch5/1 -> [VDDM_HVB4PreDet_flg]  "VDDM_HVB4PreDet_flg"
  Constant43/1 -> Timer1/4
  Constant40/1 -> Test Detection Criteria/3
  VINP_HVBattReady4Pre_enum/1 -> Equal24/1
  Constant3/1 -> Equal24/2
  task_time_s/1 -> [task_time_s]
  VPMM_PwrStaSW_enum/1 -> [VPMM_PwrStaSW_enum]
  VPMM_PowerSta_enum/1 -> [VPMM_PowerSta_enum]

== system ddm/DDM/DDM/PMM/power up and power down/High level system safety check fail ==
  note: Diagnostics and Fault Handling
  note: Release Condition After Failure Decision
  note: Test Detection Criteria
  note: Test Pass Criteria
  note: Release Condition During Failure Detection
  note: Fail Safe Operation During Failure Detection
  note: Fail Safe Operation After Failure Decision
  task_time_s : Inport
  VPMM_PowerSta_enum : Inport  Port=2
  VPMM_PwrStaSW_enum : Inport  Port=3
  VPMM_SafetyChkHLv_flg : Inport  Port=4
  VPMM_PowerUpFault_enum : Inport  Port=5
  DTC_clear_request : Inport  Port=6
  VPMM_PowerUpState_enum : Inport  Port=7
  Constant : Constant  Value=ENUM_PUFAULT_SAFETYCHKFAIL
  Constant1 : Constant  Value=ENUM_PUSTATE_COMPLETED
  Constant10 : Constant  Value=KDDM_HiLvSaChkDTC_cnt
  Constant11 : Constant  Value=KDDM_HiLvSaChkPassSW_flg
  Constant15 : Constant  Value=KDDM_HiLvSaChkCFSSW_flg
  Constant16 : Constant  Value=TRUE
  Constant19 : Constant  Value=ENUM_POWERSTA_OFF
  Constant{2,21,25,27} (4 alike) : Constant  Value=FALSE
  Constant20 : Constant  Value=KDDM_HiLvSaChkDFSSW_flg
  Constant23 : Constant  Value=TRUE
  Constant24 : Constant  Value=TRUE
  Constant26 : Constant  Value=ENUM_PWRSTASW_OFF
  Constant38 : Constant  Commented=on  Value=KDDM_HiLvSaChkDetTO_s
  Constant40 : Constant  Commented=on  Value=KDDM_HiLvSaChkDTC_cnt
  Constant43 : Constant  Value=KDDM_HiLvSaChkPassTO_s
  Constant44 : Constant  Value=KDDM_HiLvSaChkDetSW_flg
  Constant8 : Constant  Value=KDDM_HiLvSaChkPassTO_s
  DTC_Couter : hcu_lib/Basic_Blocks/DTC_Couter
  DTC_Info : hcu_lib/Basic_Blocks/DTC_Info
  Data Type Conversion1 : DataTypeConversion  OutDataTypeStr=uint8
  Equal : RelationalOperator  Operator=~=  OutDataTypeStr=boolean  RndMeth=Simplest
  Equal1 : RelationalOperator  Operator===  OutDataTypeStr=boolean  RndMeth=Simplest
  Equal2 : RelationalOperator  Operator===  OutDataTypeStr=boolean  RndMeth=Simplest
  Equal5 : RelationalOperator  OutDataTypeStr=boolean  RndMeth=Simplest
  Equal6 : RelationalOperator  Operator===  OutDataTypeStr=boolean  RndMeth=Simplest
  From48 : From  Commented=on  GotoTag=task_time_s
  Goto24 : Goto  Commented=on  GotoTag=VDDM_EDriveSysErrVCUErr_flg
  Logical Operator1 : Logic  Operator=NOT  AllPortsSameDT=off  OutDataTypeStr=boolean
  Logical Operator{5,12,15,18} (4 alike) : Logic  AllPortsSameDT=off  OutDataTypeStr=boolean
  Logical Operator19 : Logic  Inputs=3  AllPortsSameDT=off  OutDataTypeStr=boolean
  Logical Operator2 : Logic  Operator=OR  AllPortsSameDT=off  OutDataTypeStr=boolean
  Logical Operator3 : Logic  Operator=OR  Inputs=3  AllPortsSameDT=off  OutDataTypeStr=boolean
  Logical Operator4 : Logic  Operator=NOT  AllPortsSameDT=off  OutDataTypeStr=boolean
  Logical Operator6 : Logic  Operator=NOT  AllPortsSameDT=off  OutDataTypeStr=boolean
  Logical Operator7 : Logic  Operator=OR  AllPortsSameDT=off  OutDataTypeStr=boolean
  Logical Operator8 : Logic  Operator=OR  AllPortsSameDT=off  OutDataTypeStr=boolean
  Relay : Relay  OnSwitchValue=ONE_INT  OffSwitchValue=ZERO_INT
  SR_Latch1 : Subsystem  mask(SR_Latch){}
      mask help: SR latch function.
  SR_Latch3 : hcu_lib/Basic_Blocks/SR_Latch
  SR_Latch4 : hcu_lib/Basic_Blocks/SR_Latch
  Switch{,2,4..5} (4 alike) : Switch  Criteria=u2 ~= 0
  Test Detection Criteria : hcu_lib/Basic_Blocks/Test Detection Criteria  Commented=on
  Timer1 : hcu_lib/Basic_Blocks/Timer
  VDDM_HiLvSaChkDTC_raw32 : Outport
  wires:
  SR_Latch3/1 -> Logical Operator12/2
  Logical Operator2/1 -> SR_Latch4/2
  [DTC_clear_request] -> Logical Operator7/2
  [DTC_clear_request] -> Logical Operator2/2
  [VDDM_HiLvSaChkPass_flg] -> Logical Operator3/1
  Logical Operator1/1 -> Logical Operator19/3
  [DTC_clear_request] -> Logical Operator1/1
  Logical Operator7/1 -> SR_Latch3/2
  [DTC_clear_request] -> Logical Operator3/3
  Constant20/1 -> Logical Operator12/1
  Constant15/1 -> Logical Operator18/2
  Logical Operator3/1 -> Logical Operator15/1
  [VDDM_HiLvSaChkCFSRls_flg] -> Logical Operator3/2
  Logical Operator18/1 -> [VDDM_HiLvSaChkCFS_flg]  "VDDM_HiLvSaChkCFS_flg"
  Logical Operator19/1 -> DTC_Couter/1
  Constant10/1 -> DTC_Couter/3
  Constant11/1 -> Logical Operator15/2
  [VDDM_HiLvSaChkDet_flg] -> Logical Operator19/1
  SR_Latch4/1 -> Logical Operator18/1
  Logical Operator15/1 -> DTC_Couter/2
  Constant44/1 -> Logical Operator19/2
  [VDDM_HiLvSaChkCFSRls_flg] -> Logical Operator2/1
  Logical Operator12/1 -> [VDDM_HiLvSaChkDFS_flg]  "VDDM_HiLvSaChkDFS_flg"
  Relay/1 -> SR_Latch3/1
  [VDDM_HiLvSaChkDTC_cnt] -> Relay/1
  DTC_Couter/2 -> Data Type Conversion1/1
  Data Type Conversion1/1 -> [VDDM_HiLvSaChkDTC_cnt]  "VDDM_HiLvSaChkDTC_cnt"
  [VDDM_HiLvSaChkCFS_flg] -> Logical Operator7/1
  DTC_Couter/1 -> SR_Latch4/1
  [VPMM_PowerUpState_enum] -> Equal2/1
  Constant1/1 -> Equal2/2
  Constant2/1 -> Switch2/1
  VPMM_PowerUpState_enum/1 -> [VPMM_PowerUpState_enum]
  [DTC_clear_request] -> DTC_Info/4
  Constant38/1 -> Test Detection Criteria/4
  [VDDM_HiLvSaChkDet_flg] -> DTC_Info/1
  [VDDM_HiLvSaChkCFS_flg] -> DTC_Info/3
  [VDDM_HiLvSaChkPass_flg] -> DTC_Info/2
  DTC_Info/1 -> VDDM_HiLvSaChkDTC_raw32/1  "VDDM_HiLvSaChkDTC_raw32"
  task_time_s/1 -> [task_time_s]
  VPMM_PwrStaSW_enum/1 -> [VPMM_PwrStaSW_enum]
  VPMM_PowerSta_enum/1 -> [VPMM_PowerSta_enum]
  Constant21/1 -> Switch/3
  Equal5/1 -> SR_Latch1/1(set)
  Switch4/1 -> [VDDM_HiLvSaChkCFSRls_flg]  "VDDM_HiLvSaChkCFSRls_flg"
  Constant8/1 -> Equal5/2
  [task_time_s] -> Timer1/3
  [VPMM_PowerSta_enum] -> Equal6/1
  Constant23/1 -> Switch2/3
  Constant16/1 -> Switch/1
  Constant26/1 -> Equal/2
  From48/1 -> Test Detection Criteria/2
  Switch/1 -> Goto24/1
  Switch5/1 -> [VDDM_HiLvSaChkDet_flg]  "VDDM_HiLvSaChkDet_flg"
  Constant24/1 -> Switch4/1
  Constant40/1 -> Test Detection Criteria/3
  Constant25/1 -> Switch4/3
  [VPMM_PwrStaSW_enum] -> Equal/1
  [VDDM_HiLvSaChkCFS_flg] -> Switch/2
  [DTC_clear_request] -> Logical Operator8/2
  Equal2/1 -> Switch2/2
  Equal/1 -> Switch5/2
  Logical Operator8/1 -> Switch4/2
  Logical Operator6/1 -> Timer1/1
  SR_Latch1/1(latched) -> [VDDM_HiLvSaChkPass_flg]  "VDDM_HiLvSaChkPass_flg"
  Equal6/1 -> Logical Operator8/1
  Constant27/1 -> Switch5/3
  Constant43/1 -> Timer1/4
  Constant19/1 -> Equal6/2
  [VDDM_HiLvSaChkChk_flg] -> Switch5/1
  Timer1/1 -> Equal5/1
  Switch2/1 -> SR_Latch1/2(reset), Timer1/2, Logical Operator6/1
  DTC_clear_request/1 -> [DTC_clear_request]
  Constant/1 -> Equal1/2
  Equal1/1 -> Logical Operator5/2
  Logical Operator4/1 -> Logical Operator5/1
  VPMM_SafetyChkHLv_flg/1 -> Logical Operator4/1
  VPMM_PowerUpFault_enum/1 -> Equal1/1
  Logical Operator5/1 -> [VDDM_HiLvSaChkChk_flg]

== system ddm/DDM/DDM/PMM/power up and power down/MCU active discharge fail ==
  note: Diagnostics and Fault Handling
  note: Release Condition After Failure Decision
  note: Test Pass Criteria
  note: Test Detection Criteria
  note: Fail Safe Operation During Failure Detection
  note: Fail Safe Operation After Failure Decision
  note: Release Condition During Failure Detection
  task_time_s : Inport
  VPMM_PowerSta_enum : Inport  Port=2
  VPMM_PwrStaSW_enum : Inport  Port=3
  VPMM_PowerDownFault_enum : Inport  Port=4
  DTC_clear_request : Inport  Port=5
  VPMM_MCUDCBusMaxVolt_V : Inport  Port=6
  Constant : Constant  Value=ENUM_PDFAULT_MCUDISCHRG
  Constant1 : Constant  Value=ENUM_PWRSTASW_OFF
  Constant10 : Constant  Value=KDDM_MCUActDTC_cnt
  Constant11 : Constant  Value=KDDM_MCUActPassSW_flg
  Constant15 : Constant  Value=KDDM_MCUActCFSSW_flg
  Constant16 : Constant  Value=TRUE
  Constant17 : Constant  Value=KDDM_MCUActPassTO_s
  Constant2 : Constant  Value=KPMM_MCUDischrgVolt_V
  Constant20 : Constant  Value=KDDM_MCUActDFSSW_flg
  Constant21 : Constant  Value=FALSE
  Constant22 : Constant  Value=ENUM_PWRSTASW_OFF
  Constant23 : Constant  Value=TRUE
  Constant24 : Constant  Value=TRUE
  Constant25 : Constant  Value=FALSE
  Constant27 : Constant  Value=FALSE
  Constant38 : Constant  Commented=on  Value=KDDM_MCUActDetTO_s
  Constant40 : Constant  Commented=on  Value=KDDM_MCUActDTC_cnt
  Constant43 : Constant  Value=KDDM_MCUActPassTO_s
  Constant44 : Constant  Value=KDDM_MCUActDetSW_flg
  DTC_Couter : hcu_lib/Basic_Blocks/DTC_Couter
  DTC_Info : hcu_lib/Basic_Blocks/DTC_Info
  Data Type Conversion1 : DataTypeConversion  OutDataTypeStr=uint8
  Equal1 : RelationalOperator  Operator===  OutDataTypeStr=boolean  RndMeth=Simplest
  Equal10 : RelationalOperator  Operator=<=  OutDataTypeStr=boolean  RndMeth=Simplest
  Equal2 : RelationalOperator  Operator=~=  OutDataTypeStr=boolean  RndMeth=Simplest
  Equal4 : RelationalOperator  Operator=~=  OutDataTypeStr=boolean  RndMeth=Simplest
  Equal6 : RelationalOperator  OutDataTypeStr=boolean  RndMeth=Simplest
  From48 : From  Commented=on  GotoTag=task_time_s
  Logical Operator1 : Logic  Operator=NOT  AllPortsSameDT=off  OutDataTypeStr=boolean
  Logical Operator12 : Logic  AllPortsSameDT=off  OutDataTypeStr=boolean
  Logical Operator15 : Logic  AllPortsSameDT=off  OutDataTypeStr=boolean
  Logical Operator18 : Logic  AllPortsSameDT=off  OutDataTypeStr=boolean
  Logical Operator19 : Logic  Inputs=3  AllPortsSameDT=off  OutDataTypeStr=boolean
  Logical Operator2 : Logic  Operator=OR  AllPortsSameDT=off  OutDataTypeStr=boolean
  Logical Operator3 : Logic  Operator=OR  Inputs=3  AllPortsSameDT=off  OutDataTypeStr=boolean
  Logical Operator4 : Logic  Operator=OR  AllPortsSameDT=off  OutDataTypeStr=boolean
  Logical Operator6 : Logic  Operator=NOT  AllPortsSameDT=off  OutDataTypeStr=boolean
  Logical Operator8 : Logic  Operator=OR  AllPortsSameDT=off  OutDataTypeStr=boolean
  Relay : Relay  OnSwitchValue=ONE_INT  OffSwitchValue=ZERO_INT
  SR_Latch1 : Subsystem  mask(SR_Latch){}
      mask help: SR latch function.
  SR_Latch3 : hcu_lib/Basic_Blocks/SR_Latch
  SR_Latch4 : hcu_lib/Basic_Blocks/SR_Latch
  Switch{,1,4..5} (4 alike) : Switch  Criteria=u2 ~= 0
  Test Detection Criteria : hcu_lib/Basic_Blocks/Test Detection Criteria  Commented=on
  Timer1 : hcu_lib/Basic_Blocks/Timer
  VDDM_MCUActDTC_raw32 : Outport
  VDDM_MCUActDisFail_flg : Outport  Port=2
  VDDM_MCUActCFS_flg : Outport  Port=3
  wires:
  Equal10/1 -> Logical Operator8/1
  Constant2/1 -> Equal10/2
  [VPMM_MCUDCBusMaxVolt_V] -> Equal10/1
  VPMM_MCUDCBusMaxVolt_V/1 -> [VPMM_MCUDCBusMaxVolt_V]
  [VDDM_MCUActCFS_flg] -> VDDM_MCUActCFS_flg/1
  [VDDM_MCUActPass_flg] -> Logical Operator3/1
  [VDDM_MCUActCFSRls_flg] -> Logical Operator3/2
  Logical Operator4/1 -> SR_Latch3/2
  Logical Operator15/1 -> DTC_Couter/2
  Constant11/1 -> Logical Operator15/2
  [VDDM_MCUActCFSRls_flg] -> Logical Operator2/1
  DTC_Couter/1 -> SR_Latch4/1
  SR_Latch4/1 -> Logical Operator18/1
  Logical Operator2/1 -> SR_Latch4/2
  Logical Operator12/1 -> [VDDM_MCUActDFS_flg]  "VDDM_MCUActDFS_flg"
  Data Type Conversion1/1 -> [VDDM_MCUActDTC_cnt]  "VDDM_MCUActDTC_cnt"
  Logical Operator19/1 -> DTC_Couter/1
  Constant15/1 -> Logical Operator18/2
  [DTC_clear_request] -> Logical Operator1/1
  SR_Latch3/1 -> Logical Operator12/2
  [VDDM_MCUActDet_flg] -> Logical Operator19/1
  Constant20/1 -> Logical Operator12/1
  [VDDM_MCUActCFS_flg] -> Logical Operator4/1
  [DTC_clear_request] -> Logical Operator4/2
  DTC_Couter/2 -> Data Type Conversion1/1
  [VDDM_MCUActDTC_cnt] -> Relay/1
  [DTC_clear_request] -> Logical Operator2/2
  Logical Operator1/1 -> Logical Operator19/3
  Logical Operator3/1 -> Logical Operator15/1
  Constant44/1 -> Logical Operator19/2
  Relay/1 -> SR_Latch3/1
  Constant10/1 -> DTC_Couter/3
  Logical Operator18/1 -> [VDDM_MCUActCFS_flg]  "VDDM_MCUActCFS_flg"
  [DTC_clear_request] -> Logical Operator3/3
  [DTC_clear_request] -> DTC_Info/4
  Constant38/1 -> Test Detection Criteria/4
  [VDDM_MCUActDet_flg] -> DTC_Info/1
  [VDDM_MCUActCFS_flg] -> DTC_Info/3
  [VDDM_MCUActPass_flg] -> DTC_Info/2
  DTC_Info/1 -> VDDM_MCUActDTC_raw32/1  "VDDM_MCUActDTC_raw32"
  [VDDM_MCUActDisFail_flg] -> VDDM_MCUActDisFail_flg/1
  Equal1/1 -> [VDDM_MCUActChk_flg]
  VPMM_PowerDownFault_enum/1 -> Equal1/1
  Constant/1 -> Equal1/2
  DTC_clear_request/1 -> [DTC_clear_request]
  [VDDM_MCUActChk_flg] -> Switch5/1
  [VPMM_PwrStaSW_enum] -> Equal4/1
  Constant21/1 -> Switch/3
  [task_time_s] -> Timer1/3
  [VDDM_MCUActCFS_flg] -> Switch/2
  [VDDM_MCUActChk_flg] -> Switch1/1
  Constant25/1 -> Switch4/3
  Constant22/1 -> Equal4/2
  Logical Operator8/1 -> Switch4/2
  Constant43/1 -> Timer1/4
  Equal6/1 -> SR_Latch1/1(set)
  Switch1/1 -> Timer1/2, SR_Latch1/2(reset), Logical Operator6/1
  Timer1/1 -> Equal6/1
  Constant16/1 -> Switch/1
  Constant24/1 -> Switch4/1
  Switch/1 -> [VDDM_MCUActDisFail_flg]  "VDDM_MCUActDisFail_flg"
  Logical Operator6/1 -> Timer1/1
  Constant17/1 -> Equal6/2
  From48/1 -> Test Detection Criteria/2
  Switch4/1 -> [VDDM_MCUActCFSRls_flg]  "VDDM_MCUActCFSRls_flg"
  Constant40/1 -> Test Detection Criteria/3
  [DTC_clear_request] -> Logical Operator8/2
  Switch5/1 -> [VDDM_MCUActDet_flg]  "VDDM_MCUActDet_flg"
  Constant1/1 -> Equal2/2
  [VPMM_PwrStaSW_enum] -> Equal2/1
  Equal4/1 -> Switch5/2
  SR_Latch1/1(latched) -> [VDDM_MCUActPass_flg]  "VDDM_MCUActPass_flg"
  Equal2/1 -> Switch1/2
  Constant23/1 -> Switch1/3
  Constant27/1 -> Switch5/3
  task_time_s/1 -> [task_time_s]
  VPMM_PwrStaSW_enum/1 -> [VPMM_PwrStaSW_enum]
  VPMM_PowerSta_enum/1 -> [VPMM_PowerSta_enum]
